simulink model "LQR"  (R2023a)
settings: Solver=VariableStepAuto  StartTime=0.0  StopTime=10.0  RelTol=1e-3
settings Model: Creator=Wu Shidong  LastModifiedBy=Wu Shidong

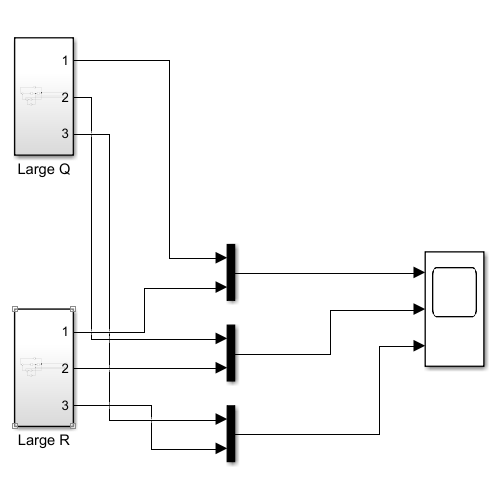
[thumbnail: Simulink's stored preview of the top-level diagram]
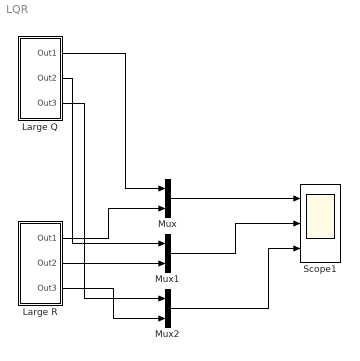
== system LQR ==
  Large Q : Subsystem
  Large R : Subsystem
  Mux : Mux  Inputs=2
  Mux1 : Mux  Inputs=2
  Mux2 : Mux  Inputs=2
  Scope1 : Scope  NumInputPorts=3
  wires:
  Large Q/2(Out2) -> Mux1/1
  Large Q/3(Out3) -> Mux2/1
  Large R/2(Out2) -> Mux1/2
  Large R/3(Out3) -> Mux2/2
  Large R/1(Out1) -> Mux/2
  Mux/1 -> Scope1/1
  Large Q/1(Out1) -> Mux/1
  Mux1/1 -> Scope1/2
  Mux2/1 -> Scope1/3

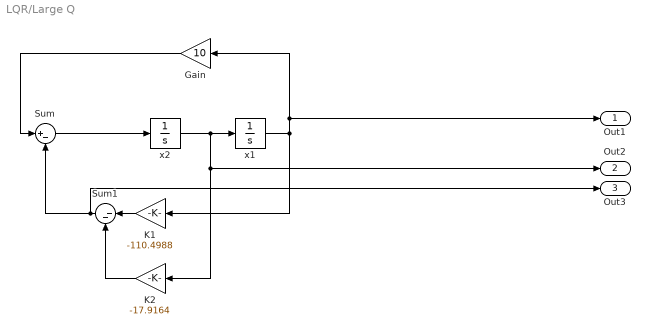
== system LQR/Large Q ==
  Gain : Gain  Gain=10
  K1 : Gain  Gain=-110.4988
  K2 : Gain  Gain=-17.9164
  Sum : Sum  Inputs=|+-
  Sum1 : Sum  Inputs=|--
  x1 : Integrator  InitialCondition=5
  x2 : Integrator
  Out1 : Outport
  Out2 : Outport  Port=2
  Out3 : Outport  Port=3
  wires:
  x1/1 -> Out1/1, Gain/1, K1/1
  Gain/1 -> Sum/1
  K1/1 -> Sum1/1
  Sum1/1 -> Out3/1, Sum/2
  Sum/1 -> x2/1
  x2/1 -> K2/1, Out2/1, x1/1
  K2/1 -> Sum1/2

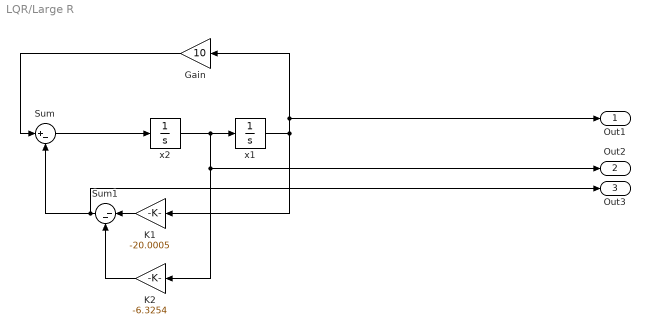
== system LQR/Large R ==
  Gain : Gain  Gain=10
  K1 : Gain  Gain=-20.0005
  K2 : Gain  Gain=-6.3254
  Sum : Sum  Inputs=|+-
  Sum1 : Sum  Inputs=|--
  x1 : Integrator  InitialCondition=5
  x2 : Integrator
  Out1 : Outport
  Out2 : Outport  Port=2
  Out3 : Outport  Port=3
  wires:
  x1/1 -> Out1/1, Gain/1, K1/1
  Gain/1 -> Sum/1
  K1/1 -> Sum1/1
  Sum1/1 -> Out3/1, Sum/2
  Sum/1 -> x2/1
  x2/1 -> K2/1, Out2/1, x1/1
  K2/1 -> Sum1/2
